simulink model "generic_20231123_1032"  (R2022b)
settings: Solver=ode45  StartTime=0.0  StopTime=50  RelTol=1e-3  EnableMultiTasking=on
model workspace (MAT data in the model file):
  A = 1
  B = 1.19071237887
  kd = -9.99955278144
  ki = 0.00519416981022
  kp = 9.99999979837
undefined symbols (not defined in the file): brake_select, curvature, DiscIntNeverNeededParam, speed
libraries: CarMaker4SL x88, simulink x1, mpcadaslib x1
(part 3 of 4)

== system generic_20231123_1032/CarMaker/IPG Vehicle/CarAndTrailer/Trailer/CreateBus Car.Hitch.FrcTrq ==
  In1 : Inport
  Bus Creator7 : BusCreator  Inputs=6
  Demux7 : Demux  Outputs=6
      settings: DisplayOption=none
  Out1 : Outport  VectorParamsAs1DForOutWhenUnconnected=off
  wires:
  In1/1 -> Demux7/1
  Bus Creator7/1 -> Out1/1
  Demux7/6 -> Bus Creator7/6  "Car Hitch Trq2Car z"
  Demux7/5 -> Bus Creator7/5  "Car Hitch Trq2Car y"
  Demux7/4 -> Bus Creator7/4  "Car Hitch Trq2Car x"
  Demux7/3 -> Bus Creator7/3  "Car Hitch Frc2Car z"
  Demux7/2 -> Bus Creator7/2  "Car Hitch Frc2Car y"
  Demux7/1 -> Bus Creator7/1  "Car Hitch Frc2Car x"

== system generic_20231123_1032/CarMaker/IPG Vehicle/CarAndTrailer/Trailer/CreateBus Vhcl.Motion ==
  In1 : Inport
  BusCreator : BusCreator  Inputs=15
  Demux : Demux  Outputs=15
      settings: DisplayOption=none
  Out1 : Outport  VectorParamsAs1DForOutWhenUnconnected=off
  wires:
  Demux/15 -> BusCreator/15  "Vhcl YawAcc"
  Demux/14 -> BusCreator/14  "Vhcl YawVel"
  Demux/13 -> BusCreator/13  "Vhcl Yaw"
  Demux/12 -> BusCreator/12  "Vhcl PitchAcc"
  Demux/11 -> BusCreator/11  "Vhcl PitchVel"
  Demux/10 -> BusCreator/10  "Vhcl Pitch"
  Demux/9 -> BusCreator/9  "Vhcl RollAcc"
  Demux/8 -> BusCreator/8  "Vhcl RollVel"
  Demux/7 -> BusCreator/7  "Vhcl Roll"
  Demux/6 -> BusCreator/6  "Vhcl Hitch_Pos z"
  Demux/5 -> BusCreator/5  "Vhcl Hitch_Pos y"
  Demux/4 -> BusCreator/4  "Vhcl Hitch_Pos x"
  Demux/3 -> BusCreator/3  "Vhcl sRoad"
  Demux/2 -> BusCreator/2  "Vhcl Distance"
  Demux/1 -> BusCreator/1  "Vhcl v"
  In1/1 -> Demux/1
  BusCreator/1 -> Out1/1

== system generic_20231123_1032/CarMaker/IPG Vehicle/CarAndTrailer/Trailer/CreateBus Vhcl.PoI ==
  In1 : Inport
  Bus Creator3 : BusCreator  Inputs=18
  Demux3 : Demux  Outputs=18
      settings: DisplayOption=none
  Out1 : Outport  VectorParamsAs1DForOutWhenUnconnected=off
  wires:
  Demux3/18 -> Bus Creator3/18  "Vhcl PoI_GCS Elev"
  Demux3/17 -> Bus Creator3/17  "Vhcl PoI_GCS Lat"
  Demux3/16 -> Bus Creator3/16  "Vhcl PoI_GCS Long"
  Demux3/15 -> Bus Creator3/15  "Vhcl PoI_Acc_1 z"
  Demux3/14 -> Bus Creator3/14  "Vhcl PoI_Acc_1 y"
  Demux3/13 -> Bus Creator3/13  "Vhcl PoI_Acc_1 x"
  Demux3/12 -> Bus Creator3/12  "Vhcl PoI_Vel_1 z"
  Demux3/11 -> Bus Creator3/11  "Vhcl PoI_Vel_1 y"
  Demux3/10 -> Bus Creator3/10  "Vhcl PoI_Vel_1 x"
  Demux3/9 -> Bus Creator3/9  "Vhcl PoI_Acc z"
  Demux3/8 -> Bus Creator3/8  "Vhcl PoI_Acc y"
  Demux3/7 -> Bus Creator3/7  "Vhcl PoI_Acc x"
  Demux3/6 -> Bus Creator3/6  "Vhcl PoI_Vel z"
  Demux3/5 -> Bus Creator3/5  "Vhcl PoI_Vel y"
  Demux3/4 -> Bus Creator3/4  "Vhcl PoI_Vel x"
  Demux3/3 -> Bus Creator3/3  "Vhcl PoI_Pos z"
  Demux3/2 -> Bus Creator3/2  "Vhcl PoI_Pos y"
  In1/1 -> Demux3/1
  Bus Creator3/1 -> Out1/1
  Demux3/1 -> Bus Creator3/1  "Vhcl PoI_Pos x"

== system generic_20231123_1032/CarMaker/IPG Vehicle/CarAndTrailer/Trailer/CreateBus Vhcl.Steering ==
  In1 : Inport
  Bus Creator3 : BusCreator  Inputs=4
  Demux : Demux
      settings: DisplayOption=none
  Out1 : Outport  VectorParamsAs1DForOutWhenUnconnected=off
  wires:
  Bus Creator3/1 -> Out1/1
  Demux/1 -> Bus Creator3/1  "Vhcl Steering Ang"
  Demux/3 -> Bus Creator3/3  "Vhcl Steering AngAcc"
  Demux/2 -> Bus Creator3/2  "Vhcl Steering AngVel"
  Demux/4 -> Bus Creator3/4  "Vhcl Steering Trq"
  In1/1 -> Demux/1

== system generic_20231123_1032/CarMaker/IPG Vehicle/CarAndTrailer/Trailer/CreateBus Vhcl.Wheel.FL ==
  In1 : Inport
  Bus Creator3 : BusCreator  Inputs=14
  Demux3 : Demux  Outputs=14
      settings: DisplayOption=none
  Out1 : Outport  VectorParamsAs1DForOutWhenUnconnected=off
  wires:
  Demux3/14 -> Bus Creator3/14  "Vhcl Wheel FL Trq_WhlBearing"
  Demux3/13 -> Bus Creator3/13  "Vhcl Wheel FL Trq_T2W"
  Demux3/12 -> Bus Creator3/12  "Vhcl Wheel FL SideSlip"
  Demux3/11 -> Bus Creator3/11  "Vhcl Wheel FL LongSlip"
  Demux3/10 -> Bus Creator3/10  "Vhcl Wheel FL vBelt"
  Demux3/9 -> Bus Creator3/9  "Vhcl Wheel FL Fz"
  Demux3/8 -> Bus Creator3/8  "Vhcl Wheel FL Fy"
  Demux3/7 -> Bus Creator3/7  "Vhcl Wheel FL Fx"
  Demux3/6 -> Bus Creator3/6  "Vhcl Wheel FL r_zxy z"
  Demux3/5 -> Bus Creator3/5  "Vhcl Wheel FL r_zxy y"
  Demux3/4 -> Bus Creator3/4  "Vhcl Wheel FL r_zxy x"
  Demux3/3 -> Bus Creator3/3  "Vhcl Wheel FL t z"
  Demux3/2 -> Bus Creator3/2  "Vhcl Wheel FL t y"
  In1/1 -> Demux3/1
  Bus Creator3/1 -> Out1/1
  Demux3/1 -> Bus Creator3/1  "Vhcl Wheel FL t x"

== system generic_20231123_1032/CarMaker/IPG Vehicle/CarAndTrailer/Trailer/CreateBus Vhcl.Wheel.FR ==
  In1 : Inport
  Bus Creator3 : BusCreator  Inputs=14
  Demux3 : Demux  Outputs=14
      settings: DisplayOption=none
  Out1 : Outport  VectorParamsAs1DForOutWhenUnconnected=off
  wires:
  Demux3/14 -> Bus Creator3/14  "Vhcl Wheel FR Trq_WhlBearing"
  Demux3/13 -> Bus Creator3/13  "Vhcl Wheel FR Trq_T2W"
  Demux3/12 -> Bus Creator3/12  "Vhcl Wheel FR SideSlip"
  Demux3/11 -> Bus Creator3/11  "Vhcl Wheel FR LongSlip"
  Demux3/10 -> Bus Creator3/10  "Vhcl Wheel FR vBelt"
  Demux3/9 -> Bus Creator3/9  "Vhcl Wheel FR Fz"
  Demux3/8 -> Bus Creator3/8  "Vhcl Wheel FR Fy"
  Demux3/7 -> Bus Creator3/7  "Vhcl Wheel FR Fx"
  Demux3/6 -> Bus Creator3/6  "Vhcl Wheel FR r_zxy z"
  Demux3/5 -> Bus Creator3/5  "Vhcl Wheel FR r_zxy y"
  Demux3/4 -> Bus Creator3/4  "Vhcl Wheel FR r_zxy x"
  Demux3/3 -> Bus Creator3/3  "Vhcl Wheel FR t z"
  Demux3/2 -> Bus Creator3/2  "Vhcl Wheel FR t y"
  In1/1 -> Demux3/1
  Bus Creator3/1 -> Out1/1
  Demux3/1 -> Bus Creator3/1  "Vhcl Wheel FR t x"

== system generic_20231123_1032/CarMaker/IPG Vehicle/CarAndTrailer/Trailer/CreateBus Vhcl.Wheel.RL ==
  In1 : Inport
  Bus Creator3 : BusCreator  Inputs=14
  Demux3 : Demux  Outputs=14
      settings: DisplayOption=none
  Out1 : Outport  VectorParamsAs1DForOutWhenUnconnected=off
  wires:
  Demux3/14 -> Bus Creator3/14  "Vhcl Wheel RL Trq_WhlBearing"
  Demux3/13 -> Bus Creator3/13  "Vhcl Wheel RL Trq_T2W"
  Demux3/12 -> Bus Creator3/12  "Vhcl Wheel RL SideSlip"
  Demux3/11 -> Bus Creator3/11  "Vhcl Wheel RL LongSlip"
  Demux3/10 -> Bus Creator3/10  "Vhcl Wheel RL vBelt"
  Demux3/9 -> Bus Creator3/9  "Vhcl Wheel RL Fz"
  Demux3/8 -> Bus Creator3/8  "Vhcl Wheel RL Fy"
  Demux3/7 -> Bus Creator3/7  "Vhcl Wheel RL Fx"
  Demux3/6 -> Bus Creator3/6  "Vhcl Wheel RL r_zxy z"
  Demux3/5 -> Bus Creator3/5  "Vhcl Wheel RL r_zxy y"
  Demux3/4 -> Bus Creator3/4  "Vhcl Wheel RL r_zxy x"
  Demux3/3 -> Bus Creator3/3  "Vhcl Wheel RL t z"
  Demux3/2 -> Bus Creator3/2  "Vhcl Wheel RL t y"
  In1/1 -> Demux3/1
  Bus Creator3/1 -> Out1/1
  Demux3/1 -> Bus Creator3/1  "Vhcl Wheel RL t x"

== system generic_20231123_1032/CarMaker/IPG Vehicle/CarAndTrailer/Trailer/CreateBus Vhcl.Wheel.RR ==
  In1 : Inport
  Bus Creator3 : BusCreator  Inputs=14
  Demux3 : Demux  Outputs=14
      settings: DisplayOption=none
  Out1 : Outport  VectorParamsAs1DForOutWhenUnconnected=off
  wires:
  Demux3/14 -> Bus Creator3/14  "Vhcl Wheel RR Trq_WhlBearing"
  Demux3/13 -> Bus Creator3/13  "Vhcl Wheel RR Trq_T2W"
  Demux3/12 -> Bus Creator3/12  "Vhcl Wheel RR SideSlip"
  Demux3/11 -> Bus Creator3/11  "Vhcl Wheel RR LongSlip"
  Demux3/10 -> Bus Creator3/10  "Vhcl Wheel RR vBelt"
  Demux3/9 -> Bus Creator3/9  "Vhcl Wheel RR Fz"
  Demux3/8 -> Bus Creator3/8  "Vhcl Wheel RR Fy"
  Demux3/7 -> Bus Creator3/7  "Vhcl Wheel RR Fx"
  Demux3/6 -> Bus Creator3/6  "Vhcl Wheel RR r_zxy z"
  Demux3/5 -> Bus Creator3/5  "Vhcl Wheel RR r_zxy y"
  Demux3/4 -> Bus Creator3/4  "Vhcl Wheel RR r_zxy x"
  Demux3/3 -> Bus Creator3/3  "Vhcl Wheel RR t z"
  Demux3/2 -> Bus Creator3/2  "Vhcl Wheel RR t y"
  In1/1 -> Demux3/1
  Bus Creator3/1 -> Out1/1
  Demux3/1 -> Bus Creator3/1  "Vhcl Wheel RR t x"

== system generic_20231123_1032/CarMaker/VehicleControl/CreateBus VhclCtrl/Stanley_controller/Stanley ==
  Path_out : Inport
  <Vx_Global_m_s> : Inport  Port=2
  <Vy_Global_m_s> : Inport  Port=3
  <Yaw_angle_rad> : Inport  Port=4
  <Actual_Velocity_Car_m_s> : Inport  Port=5
  Desired_speed : Inport  Port=6
  Actual velocity [km/h] : Display
  Bus Selector : BusSelector  OutputSignals=Path.tx,Path.ty
  Constant1 : Constant  Value=0
  Delay : Delay  DelayLength=1
  Delay1 : Delay  DelayLength=1
  Gain : Gain  Gain=3.6
  Read CM Dict : CarMaker4SL/Read CM Dict  xname=Car.Road.Path.DevDist  xsync=off  xstime=Continuous
  Read CM Dict1 : CarMaker4SL/Read CM Dict  xname=Car.Con.tx  xsync=off  xstime=Continuous
  Read CM Dict2 : CarMaker4SL/Read CM Dict  xname=Car.Con.ty  xsync=off  xstime=Continuous
  Road Sensor : CarMaker4SL/Sensors/Road Sensor  xname=0  xstime=Continuous
      settings: SourceProductName=CarMaker4SL
  Saturation : Saturate  UpperLimit=pi()/6  LowerLimit=-pi/6
  Scope : Scope  NumInputPorts=3
  Smoothing : Subsystem
  Stanely_controller : MATLAB Function  TreatAsAtomicUnit=on
  Subsystem : Subsystem
  Subsystem1 : Subsystem
  Target_Steering_angle_rad : Outport  VectorParamsAs1DForOutWhenUnconnected=off
  Throttle : Outport  Port=2
  Brake_command : Outport  Port=3
  wires:
  Smoothing/1(Signal_Out) -> Target_Steering_angle_rad/1, Scope/3
  Saturation/1 -> Smoothing/1(Signal_In)  "Control signal"
  Subsystem/4(min_safe_speed) -> Subsystem1/3(min_safe_speed)
  Subsystem/2(Brake_command) -> Brake_command/1
  Subsystem/3(path_curvature) -> Subsystem1/2(curvature)
  Gain/1 -> Actual velocity [km/h]/1  "Actual velocity [km/h]"
  Stanely_controller/1(e) -> Scope/1  "Control cross track error [m]"
  <Actual_Velocity_Car_m_s>/1 -> Gain/1, Subsystem/2(speed_act), Stanely_controller/8(speed_act)
  Subsystem1/1(Target_speed) -> Subsystem/5(desired_speed)
  <Vx_Global_m_s>/1 -> Subsystem/3(velocity_x)
  <Vy_Global_m_s>/1 -> Subsystem/4(velocity_y)
  Path_out/1 -> Subsystem/1(path)
  Desired_speed/1 -> Subsystem1/1(desired_speed)
  Stanely_controller/7(steering) -> Subsystem/6(steering), Saturation/1  "steering"
  Subsystem/1(Throttle) -> Throttle/1
  Stanely_controller/6(heading_err) -> ?  "heading_error"
  Stanely_controller/2(a) -> ?  "Error [m]"
  Stanely_controller/3(b) -> ?
  Bus Selector/1 -> Stanely_controller/4(x2), Delay/1  "<tx>"
  Constant1/1 -> Road Sensor/1
  Road Sensor/2 -> Bus Selector/1
  Bus Selector/2 -> Stanely_controller/6(y2), Delay1/1  "<ty>"
  Delay1/1 -> Stanely_controller/5(y1)
  <Yaw_angle_rad>/1 -> Stanely_controller/7(yaw)  "Yaw [rad]"
  Delay/1 -> Stanely_controller/3(x1)
  Read CM Dict1/1 -> Stanely_controller/1(x_car)
  Read CM Dict/1 -> Stanely_controller/2(dev), Scope/2  "Dev_dis"

== system generic_20231123_1032/CarMaker/VehicleControl/CreateBus VhclCtrl/Subsystem1/Smoothing ==
  Signal_In : Inport
  Add : Sum  Inputs=++++
  Delay : Delay  InitialCondition=0.1
  Delay1 : Delay  DelayLength=4  InitialCondition=0.1
  Delay2 : Delay  DelayLength=5  InitialCondition=0.1
  Gain : Gain  Gain=0.35
  Gain1 : Gain  Gain=0.25
  Gain2 : Gain  Gain=0.25
  Gain3 : Gain  Gain=0.15
  Signal_Out : Outport  VectorParamsAs1DForOutWhenUnconnected=off
  wires:
  Gain1/1 -> Add/2
  Signal_In/1 -> Gain/1
  Delay/1 -> Gain1/1
  Gain/1 -> Add/1
  Delay1/1 -> Gain2/1
  Add/1 -> Delay2/1, Delay1/1, Delay/1, Signal_Out/1
  Gain2/1 -> Add/3
  Delay2/1 -> Gain3/1
  Gain3/1 -> Add/4

== system generic_20231123_1032/CarMaker/VehicleControl/CreateBus VhclCtrl/Subsystem4/Subsystem ==
  In1 : Inport
  Add : Sum  Inputs=+++
  Derivative : Derivative
  Discrete-Time Integrator : DiscreteIntegrator  SampleTime=-1  ICPrevOutput=DiscIntNeverNeededParam  ICPrevScaledInput=DiscIntNeverNeededParam
  Gain : Gain  Gain=0.6
  Gain1 : Gain  Gain=1.2
  Gain2 : Gain  Gain=0.4
  Signal_In : Outport
  wires:
  Gain1/1 -> Discrete-Time Integrator/1
  Gain2/1 -> Derivative/1
  Discrete-Time Integrator/1 -> Add/1
  Derivative/1 -> Add/3
  Gain/1 -> Add/2
  In1/1 -> Gain/1, Gain2/1, Gain1/1
  Add/1 -> Signal_In/1

== system generic_20231123_1032/CarMaker/VehicleControl/CreateBus VhclCtrl/path_planner_MATLAB/X_Global_Pos_m ==
  In1 : Inport
  Pos_X : Outport  VectorParamsAs1DForOutWhenUnconnected=off
  wires:
  In1/1 -> Pos_X/1

== system generic_20231123_1032/CarMaker/VehicleControl/CreateBus VhclCtrl/path_planner_MATLAB/Y_Global_Pos_m ==
  In1 : Inport
  Pos_Y : Outport  VectorParamsAs1DForOutWhenUnconnected=off
  wires:
  In1/1 -> Pos_Y/1

== system generic_20231123_1032/CarMaker/VehicleControl/CreateBus VhclCtrl/path_planner_MATLAB/Yaw_angle_rad ==
  In1 : Inport
  Yaw_Angle : Outport  VectorParamsAs1DForOutWhenUnconnected=off
  wires:
  In1/1 -> Yaw_Angle/1

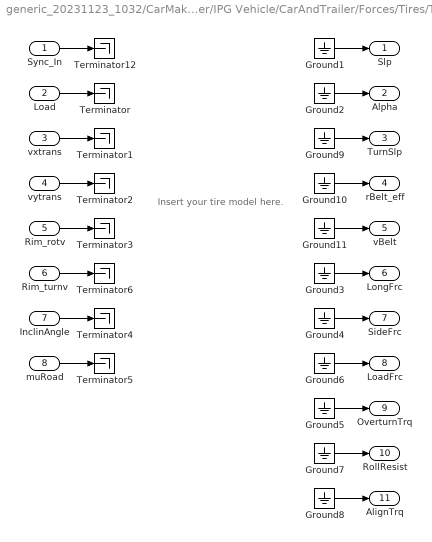
== system generic_20231123_1032/CarMaker/IPG Vehicle/CarAndTrailer/Forces/Tires/TireFL ==
  note: Insert your tire model here.
  Sync_In : Inport
  Load : Inport  Port=2
  vxtrans : Inport  Port=3
  vytrans : Inport  Port=4
  Rim_rotv : Inport  Port=5
  Rim_turnv : Inport  Port=6
  InclinAngle : Inport  Port=7
  muRoad : Inport  Port=8
  Ground{1..11} (11 alike) : Ground
  Terminator{,1..6,12} (8 alike) : Terminator
  Slp : Outport  VectorParamsAs1DForOutWhenUnconnected=off
  Alpha : Outport  Port=2  VectorParamsAs1DForOutWhenUnconnected=off
  TurnSlp : Outport  Port=3  VectorParamsAs1DForOutWhenUnconnected=off
  rBelt_eff : Outport  Port=4  VectorParamsAs1DForOutWhenUnconnected=off
  vBelt : Outport  Port=5  VectorParamsAs1DForOutWhenUnconnected=off
  LongFrc : Outport  Port=6  VectorParamsAs1DForOutWhenUnconnected=off
  SideFrc : Outport  Port=7  VectorParamsAs1DForOutWhenUnconnected=off
  LoadFrc : Outport  Port=8  VectorParamsAs1DForOutWhenUnconnected=off
  OverturnTrq : Outport  Port=9  VectorParamsAs1DForOutWhenUnconnected=off
  RollResist : Outport  Port=10  VectorParamsAs1DForOutWhenUnconnected=off
  AlignTrq : Outport  Port=11  VectorParamsAs1DForOutWhenUnconnected=off
  wires:
  Ground11/1 -> vBelt/1
  Ground10/1 -> rBelt_eff/1
  Ground9/1 -> TurnSlp/1
  Rim_turnv/1 -> Terminator6/1
  Sync_In/1 -> Terminator12/1
  Ground2/1 -> Alpha/1
  Ground3/1 -> LongFrc/1
  Ground4/1 -> SideFrc/1
  Ground5/1 -> OverturnTrq/1
  vxtrans/1 -> Terminator1/1
  vytrans/1 -> Terminator2/1
  Rim_rotv/1 -> Terminator3/1
  InclinAngle/1 -> Terminator4/1
  muRoad/1 -> Terminator5/1
  Load/1 -> Terminator/1
  Ground1/1 -> Slp/1
  Ground6/1 -> LoadFrc/1
  Ground7/1 -> RollResist/1
  Ground8/1 -> AlignTrq/1

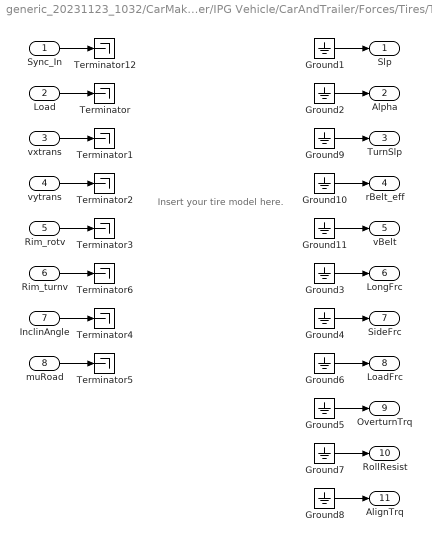
== system generic_20231123_1032/CarMaker/IPG Vehicle/CarAndTrailer/Forces/Tires/TireFR ==
  note: Insert your tire model here.
  Sync_In : Inport
  Load : Inport  Port=2
  vxtrans : Inport  Port=3
  vytrans : Inport  Port=4
  Rim_rotv : Inport  Port=5
  Rim_turnv : Inport  Port=6
  InclinAngle : Inport  Port=7
  muRoad : Inport  Port=8
  Ground{1..11} (11 alike) : Ground
  Terminator{,1..6,12} (8 alike) : Terminator
  Slp : Outport  VectorParamsAs1DForOutWhenUnconnected=off
  Alpha : Outport  Port=2  VectorParamsAs1DForOutWhenUnconnected=off
  TurnSlp : Outport  Port=3  VectorParamsAs1DForOutWhenUnconnected=off
  rBelt_eff : Outport  Port=4  VectorParamsAs1DForOutWhenUnconnected=off
  vBelt : Outport  Port=5  VectorParamsAs1DForOutWhenUnconnected=off
  LongFrc : Outport  Port=6  VectorParamsAs1DForOutWhenUnconnected=off
  SideFrc : Outport  Port=7  VectorParamsAs1DForOutWhenUnconnected=off
  LoadFrc : Outport  Port=8  VectorParamsAs1DForOutWhenUnconnected=off
  OverturnTrq : Outport  Port=9  VectorParamsAs1DForOutWhenUnconnected=off
  RollResist : Outport  Port=10  VectorParamsAs1DForOutWhenUnconnected=off
  AlignTrq : Outport  Port=11  VectorParamsAs1DForOutWhenUnconnected=off
  wires:
  Ground11/1 -> vBelt/1
  Ground10/1 -> rBelt_eff/1
  Ground9/1 -> TurnSlp/1
  Rim_turnv/1 -> Terminator6/1
  Sync_In/1 -> Terminator12/1
  Ground2/1 -> Alpha/1
  Ground3/1 -> LongFrc/1
  Ground4/1 -> SideFrc/1
  Ground5/1 -> OverturnTrq/1
  vxtrans/1 -> Terminator1/1
  vytrans/1 -> Terminator2/1
  Rim_rotv/1 -> Terminator3/1
  InclinAngle/1 -> Terminator4/1
  muRoad/1 -> Terminator5/1
  Load/1 -> Terminator/1
  Ground1/1 -> Slp/1
  Ground6/1 -> LoadFrc/1
  Ground7/1 -> RollResist/1
  Ground8/1 -> AlignTrq/1

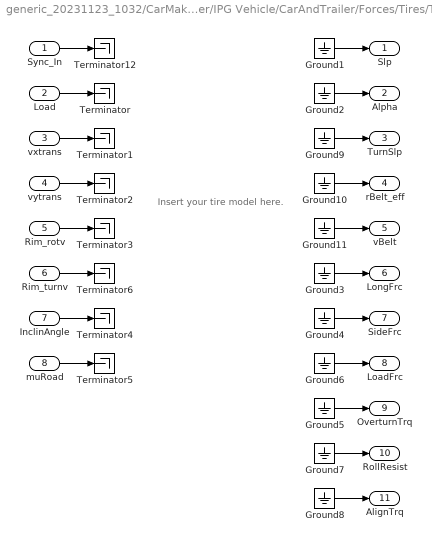
== system generic_20231123_1032/CarMaker/IPG Vehicle/CarAndTrailer/Forces/Tires/TireRL ==
  note: Insert your tire model here.
  Sync_In : Inport
  Load : Inport  Port=2
  vxtrans : Inport  Port=3
  vytrans : Inport  Port=4
  Rim_rotv : Inport  Port=5
  Rim_turnv : Inport  Port=6
  InclinAngle : Inport  Port=7
  muRoad : Inport  Port=8
  Ground{1..11} (11 alike) : Ground
  Terminator{,1..6,12} (8 alike) : Terminator
  Slp : Outport  VectorParamsAs1DForOutWhenUnconnected=off
  Alpha : Outport  Port=2  VectorParamsAs1DForOutWhenUnconnected=off
  TurnSlp : Outport  Port=3  VectorParamsAs1DForOutWhenUnconnected=off
  rBelt_eff : Outport  Port=4  VectorParamsAs1DForOutWhenUnconnected=off
  vBelt : Outport  Port=5  VectorParamsAs1DForOutWhenUnconnected=off
  LongFrc : Outport  Port=6  VectorParamsAs1DForOutWhenUnconnected=off
  SideFrc : Outport  Port=7  VectorParamsAs1DForOutWhenUnconnected=off
  LoadFrc : Outport  Port=8  VectorParamsAs1DForOutWhenUnconnected=off
  OverturnTrq : Outport  Port=9  VectorParamsAs1DForOutWhenUnconnected=off
  RollResist : Outport  Port=10  VectorParamsAs1DForOutWhenUnconnected=off
  AlignTrq : Outport  Port=11  VectorParamsAs1DForOutWhenUnconnected=off
  wires:
  Ground11/1 -> vBelt/1
  Ground10/1 -> rBelt_eff/1
  Ground9/1 -> TurnSlp/1
  Rim_turnv/1 -> Terminator6/1
  Sync_In/1 -> Terminator12/1
  Ground2/1 -> Alpha/1
  Ground3/1 -> LongFrc/1
  Ground4/1 -> SideFrc/1
  Ground5/1 -> OverturnTrq/1
  vxtrans/1 -> Terminator1/1
  vytrans/1 -> Terminator2/1
  Rim_rotv/1 -> Terminator3/1
  InclinAngle/1 -> Terminator4/1
  muRoad/1 -> Terminator5/1
  Load/1 -> Terminator/1
  Ground1/1 -> Slp/1
  Ground6/1 -> LoadFrc/1
  Ground7/1 -> RollResist/1
  Ground8/1 -> AlignTrq/1

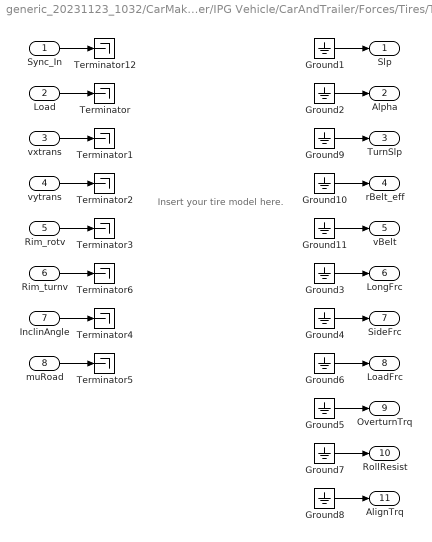
== system generic_20231123_1032/CarMaker/IPG Vehicle/CarAndTrailer/Forces/Tires/TireRR ==
  note: Insert your tire model here.
  Sync_In : Inport
  Load : Inport  Port=2
  vxtrans : Inport  Port=3
  vytrans : Inport  Port=4
  Rim_rotv : Inport  Port=5
  Rim_turnv : Inport  Port=6
  InclinAngle : Inport  Port=7
  muRoad : Inport  Port=8
  Ground{1..11} (11 alike) : Ground
  Terminator{,1..6,12} (8 alike) : Terminator
  Slp : Outport  VectorParamsAs1DForOutWhenUnconnected=off
  Alpha : Outport  Port=2  VectorParamsAs1DForOutWhenUnconnected=off
  TurnSlp : Outport  Port=3  VectorParamsAs1DForOutWhenUnconnected=off
  rBelt_eff : Outport  Port=4  VectorParamsAs1DForOutWhenUnconnected=off
  vBelt : Outport  Port=5  VectorParamsAs1DForOutWhenUnconnected=off
  LongFrc : Outport  Port=6  VectorParamsAs1DForOutWhenUnconnected=off
  SideFrc : Outport  Port=7  VectorParamsAs1DForOutWhenUnconnected=off
  LoadFrc : Outport  Port=8  VectorParamsAs1DForOutWhenUnconnected=off
  OverturnTrq : Outport  Port=9  VectorParamsAs1DForOutWhenUnconnected=off
  RollResist : Outport  Port=10  VectorParamsAs1DForOutWhenUnconnected=off
  AlignTrq : Outport  Port=11  VectorParamsAs1DForOutWhenUnconnected=off
  wires:
  Ground11/1 -> vBelt/1
  Ground10/1 -> rBelt_eff/1
  Ground9/1 -> TurnSlp/1
  Rim_turnv/1 -> Terminator6/1
  Sync_In/1 -> Terminator12/1
  Ground2/1 -> Alpha/1
  Ground3/1 -> LongFrc/1
  Ground4/1 -> SideFrc/1
  Ground5/1 -> OverturnTrq/1
  vxtrans/1 -> Terminator1/1
  vytrans/1 -> Terminator2/1
  Rim_rotv/1 -> Terminator3/1
  InclinAngle/1 -> Terminator4/1
  muRoad/1 -> Terminator5/1
  Load/1 -> Terminator/1
  Ground1/1 -> Slp/1
  Ground6/1 -> LoadFrc/1
  Ground7/1 -> RollResist/1
  Ground8/1 -> AlignTrq/1

== system generic_20231123_1032/CarMaker/VehicleControl/CreateBus VhclCtrl/Stanley_controller/Stanley/Smoothing ==
  Signal_In : Inport
  Add : Sum  Inputs=++++
  Delay : Delay  InitialCondition=0.1
  Delay1 : Delay  DelayLength=4  InitialCondition=0.1
  Delay2 : Delay  DelayLength=5  InitialCondition=0.1
  Gain : Gain  Gain=0.35
  Gain1 : Gain  Gain=0.25
  Gain2 : Gain  Gain=0.25
  Gain3 : Gain  Gain=0.15
  Signal_Out : Outport  VectorParamsAs1DForOutWhenUnconnected=off
  wires:
  Gain1/1 -> Add/2
  Signal_In/1 -> Gain/1
  Delay/1 -> Gain1/1
  Gain/1 -> Add/1
  Delay1/1 -> Gain2/1
  Add/1 -> Delay2/1, Delay1/1, Delay/1, Signal_Out/1
  Gain2/1 -> Add/3
  Delay2/1 -> Gain3/1
  Gain3/1 -> Add/4

== system generic_20231123_1032/CarMaker/VehicleControl/CreateBus VhclCtrl/Stanley_controller/Stanley/Subsystem ==
  path : Inport
  speed_act : Inport  Port=2
  velocity_x : Inport  Port=3
  velocity_y : Inport  Port=4
  desired_speed : Inport  Port=5
  steering : Inport  Port=6
  Constant : Constant  Value=0
  Constant1 : Constant  Value=kd
  Constant2 : Constant  Value=ki
  Constant3 : Constant  Value=kp
  Gain : Gain  Gain=1/1000
  Gain1 : Gain  Gain=1/1000
  Saturation : Saturate  UpperLimit=1  LowerLimit=-1
  Saturation1 : Saturate  UpperLimit=1  LowerLimit=0
  Scope : Scope  NumInputPorts=2
  advanced_speed_and_brake_control : MATLAB Function  TreatAsAtomicUnit=on
  calculate_path_curvature : MATLAB Function  TreatAsAtomicUnit=on
  Throttle : Outport
  Brake_command : Outport  Port=2
  path_curvature : Outport  Port=3
  min_safe_speed : Outport  Port=4
  wires:
  Saturation/1 -> Scope/2, Throttle/1
  Saturation1/1 -> Brake_command/1  "Brake_command"
  advanced_speed_and_brake_control/2(brake_cmd) -> Gain1/1  "Brake cmd"
  advanced_speed_and_brake_control/1(throttle) -> Gain/1  "throttle"
  desired_speed/1 -> advanced_speed_and_brake_control/4(desired_speed)
  speed_act/1 -> advanced_speed_and_brake_control/3(speed_act)
  Constant/1 -> advanced_speed_and_brake_control/1(path_curv)
  calculate_path_curvature/2(min_safe_speed) -> min_safe_speed/1, advanced_speed_and_brake_control/2(min_s_speed)
  steering/1 -> calculate_path_curvature/4(steering_angel)
  calculate_path_curvature/1(path_curvature) -> path_curvature/1
  velocity_x/1 -> calculate_path_curvature/3(velocity_x)
  velocity_y/1 -> calculate_path_curvature/2(velocity_y)
  path/1 -> calculate_path_curvature/1(path)
  Gain/1 -> Scope/1, Saturation/1
  Gain1/1 -> Saturation1/1
  Constant1/1 -> advanced_speed_and_brake_control/5(Kd_speed)
  Constant2/1 -> advanced_speed_and_brake_control/6(Ki_speed)
  Constant3/1 -> advanced_speed_and_brake_control/7(Kp_speed)

== system generic_20231123_1032/CarMaker/VehicleControl/CreateBus VhclCtrl/Stanley_controller/Stanley/Subsystem1 ==
  desired_speed : Inport
  curvature : Inport  Port=2
  min_safe_speed : Inport  Port=3
  2-D Lookup Table : Lookup_n-D  BreakpointsForDimension1=speed  BreakpointsForDimension2=curvature  Table=brake_select  InternalRulePriority=Speed  RndMeth=Simplest
      settings: InputPortMap=u0,u1
  Divide : Product  Inputs=*/
  MATLAB Function : MATLAB Function  Commented=on  TreatAsAtomicUnit=on
  Read CM Dict : CarMaker4SL/Read CM Dict  xname=Sensor.Road.VehSensor_0.Path.CurveXY  xsync=off  xstime=Continuous
  Scope2 : Scope
  Target_speed : Outport
  curv : Outport  Port=2
  speed : Outport  Port=3
  wires:
  Divide/1 -> speed/1, Target_speed/1, Scope2/1
  2-D Lookup Table/1 -> Divide/2
  desired_speed/1 -> 2-D Lookup Table/1, Divide/1
  min_safe_speed/1 -> MATLAB Function/2(min_safe_speed)
  curvature/1 -> MATLAB Function/1(u)
  Read CM Dict/1 -> curv/1, 2-D Lookup Table/2

== matlab function generic_20231123_1032/CarMaker/VehicleControl/Stanley controller/calculate_path_curvature ==
  data: path_x input; path_curvature output; path_y input
function path_curvature = calculate_path_curvature(path_x,path_y)
    x = path_x;
    y = path_y;
    % First and second derivatives
    dx = gradient(x);
    dy = gradient(y);
    
    ddx = gradient(dx);
    ddy = gradient(dy);
    
    % Path curvature
    path_curvature = mean((dx .* ddy - dy .* ddx) ./ (dx.^2 + dy.^2).^(3/2));
    %R = sqrt(1.61^2 +(1.61+1.28)^2*cot(steering_angel)^2)/12;
    
end

== matlab function generic_20231123_1032/CarMaker/VehicleControl/Stanley controller/MATLAB Function ==
  data: path input; dev input; e output; yaw input; speed_act input; err_fr_axle output; cross_track_steering output; heading_err output; steering output
function [e, err_fr_axle, cross_track_steering, heading_err, steering]  = conversion(path,dev,yaw,speed_act)
%path = [path_x;path_y];
function distance = calc_distance(pt,v1,v2)
    vect = v1 - v2;
    p_to_vect = pt - v2;
    crossVP = cross(vect,p_to_vect);
    distance = norm(crossVP) / norm(vect) * crossVP(3)/abs(crossVP(3));
end

e = zeros(1);
cross_track_steering = zeros(1);
heading_err = zeros(1);
steering=zeros(1);
err_fr_axle = zeros(1);

k_exp = 1.3059;
k = 15.028 + speed_act^k_exp;
k_ref = 2.62;

% path_index = fix(k_path * speed_act);
% if path_index > 13
%     path_index = 13;
% end
% 
% P_prev = path(:,6 + path_index);
% P_next = path(:,7 + path_index);

fr_axle = [-1.488 0 0];
distances = sqrt((path(1,:) - 1.488).^2 + (path(2,:) - 0).^2);
% Find the index of the closest point on the path
[~,err_fr_axle_ind] = min(distances);
if err_fr_axle_ind == 1
    err_fr_axle_ind = 2;
end
err_fr_axle = calc_distance(fr_axle,[path(1,err_fr_axle_ind - 1) path(2,err_fr_axle_ind - 1) 0],[path(1,err_fr_axle_ind) path(2,err_fr_axle_ind) 0]);

B = [-1.488 + k_ref * (speed_act / 27) 0 0];
distances_err = sqrt((path(1,:) - B(1)).^2 + (path(2,:) - 0).^2);
[~,err_ind] = min(distances_err);
if err_ind < 2
    err_ind = 2;
end
error = calc_distance(B,[path(1,err_ind - 1) path(2,err_ind - 1) 0],[path(1,err_ind) path(2,err_ind) 0]);


P_prev = path(:, err_ind-1);
P_next = path(:, err_ind);

x1 = P_prev(1,1);
y1 = P_prev(2,1);
x2 = P_next(1,1);
y2 = P_next(2,1);

a = (y2 - y1)/-(x2 + x1);
b = 1;
%c = -x1 * (y2 - y1) + y1 * (x2 - x1);


if speed_act ~= 0
    %e = c+b*y1/sqrt((a^2)+(b^2));
    e = error;
    
    cross_track_steering = atan(k * e / speed_act);
    heading_err = atan(-a / b) - yaw;
    %heading_err = 1/(tan(-a/b))-yaw;
    steering = heading_err + cross_track_steering;
end
end

== matlab function generic_20231123_1032/CarMaker/VehicleControl/CreateBus VhclCtrl/Subsystem1/MATLAB Function1 ==
  data: dev input; steering output; B input
function steering = advanced_speed_control_mpc(dev,B)
    % Model Predictive Controller (MPC) for speed contol
    % Define MPC parameters
    Ts = 0.1;  % Sampling time
    N = 10;    % Prediction horizon
    Q = 1;     % State weight
    R = 1;     % Input weight
    S = 0.1;   % Terminal state weight (integral term)
    
    % State-space model (simplified for illustration)
    %A = 0.8;
    %B = Ts;
    
    % Define cost and constraints for fmincon
    costFunction = @(u) (dev + B * u)' * Q * (dev + B * u) + u' * R * u + S * sum(u);
    Aeq = [];
    Beq = [];
    Aineq = [];
    Bineq = [];
    lb = -3.14; % Lower bound on throttle
    ub = 3.14;  % Upper bound on throttle
    
    % Steady-state error constraint
    Aineq = [Aineq; B];
    Bineq = [Bineq; -dev];
    
    % Initial guess
    u0 = 0;
    
    % Solve optimization problem
    options = optimoptions('fmincon', 'Display', 'off', 'Algorithm', 'sqp');
    u_opt = fmincon(costFunction, u0, Aineq, Bineq, Aeq, Beq, lb, ub, [], options);
    
    % Extract control input (throttle) from the optimization result
    steering = u_opt;
end

== matlab function generic_20231123_1032/CarMaker/VehicleControl/CreateBus VhclCtrl/Stanley_controller/Stanley/Subsystem/calculate_path_curvature ==
  data: path input; path_curvature output size=[1 20]; min_safe_speed output size=[1 20]; velocity_y input; velocity_x input; steering_angel input
function [path_curvature, min_safe_speed] = calculate_path_curvature(path,velocity_y,velocity_x,steering_angel)
    v_x = velocity_x* ones(1,20);
    v_y = velocity_y*ones(1,20);
    x = path(1,:)+v_x;
    y = path(2,:)+v_y;
    % First and second derivatives
    dx = gradient(x);
    dy = gradient(y);
    
    ddx = gradient(dx);
    ddy = gradient(dy);
    
    % Path curvature
    path_curvature = (dx .* ddy - dy .* ddx) ./ (dx.^2 + dy.^2).^(3/2);
    R = sqrt(1.61^2 +(1.61+1.28)^2*cot(steering_angel)^2)/12;
    % Minimum safe speed
    g = 9.81; % gravitational acceleration
    if max(path_curvature)>0.001 || max(path_curvature)<-0.001

        min_safe_speed = sqrt(g ./ abs(path_curvature));
    else
        min_safe_speed = sqrt(g .* abs(path_curvature));
end

== matlab function generic_20231123_1032/CarMaker/VehicleControl/CreateBus VhclCtrl/Stanley_controller/Stanley/Stanely_controller ==
  data: x_car input; dev input; x1 input; x2 input; y1 input; y2 input; yaw input; speed_act input; e output; a output; b output; c output; cross_track_steering output; heading_err output; steering output; distances output
function [e, a,b,c, cross_track_steering, heading_err, steering,distances]  = conversion(x_car,dev, x1,x2,y1,y2,yaw,speed_act)


e = zeros(1);
cross_track_steering = zeros(1);
heading_err = zeros(1);
steering=zeros(1);
err_fr_axle = zeros(1);
distances = [0 0 0 0 0 0 0 0 0 0 0 0 0 0 0 0 0 0 0 0];

k_exp = 1.36;
k_def = 6;
k = k_def + abs(speed_act)^k_exp;
k_ref = 3.1;



% Perform linear regression to find a, b, and c
% X = [path(1, :); path(2, :); ones(1, 20)]';  % Create a matrix for linear regression
% coefficients = X \ -1 * ones(20, 1);
% 
% % Extract the coefficients a, b, and c
% a = coefficients(1);
% b = coefficients(2);
% c = coefficients(3);



%Trajectory line ax+by+c = 0
% OR y= slope *x +y_intercept
% slope = path(2,)% [2-20]
if (x2 ==0 && x1 ==0)|| x2==x1
a = 0;
b = 1;
c = y2+a*x2;
else
a = -(y2 - y1)/(x2-x1);
b = 1;
c = y2+a*x2;
end

if speed_act ~=0
    %e =abs(a*x_car+b*y_car+c)\sqrt(a^2+b^2); %abs(Dev_dis);
    e =abs(dev);
    cross_track_steering = atan(e*k / speed_act);

    heading_err = atan(-a/b)-yaw;
    steering = heading_err + cross_track_steering;

else
    steering = 0;
end
end

== matlab function generic_20231123_1032/CarMaker/VehicleControl/CreateBus VhclCtrl/Subsystem1/MATLAB Function2 ==
  data: x_car input; target_heading output; y_car input; x_path input; y_path input; yaw_angle input; current_heading output
function [target_heading, current_heading] = calculate_headings(x_car, y_car, x_path, y_path, yaw_angle)
    % Calculate headings based on car and path positions and yaw angle
    function angle = normalize_angle(angle)
    % Normalize an angle to be in the range [-pi, pi]
    while angle > pi
        angle = angle - 2*pi;
    end

    while angle < -pi
        angle = angle + 2*pi;
    end
end
    % Calculate angle from car to path (target_heading)
    target_heading = atan2(y_path - y_car, x_path - x_car);
    
    % Adjust yaw angle to be in the range [-pi, pi]
    yaw_angle = normalize_angle(yaw_angle);
    
    % Current heading is the yaw angle of the vehicle
    current_heading = yaw_angle;
end

== matlab function generic_20231123_1032/CarMaker/VehicleControl/CreateBus VhclCtrl/Stanley_controller/Stanley/Subsystem1/MATLAB Function ==
  data: u input; curv output; min_safe_speed input; speed output
function [curv, speed] = fcn(u, min_safe_speed)

curv = abs(max(u));
speed = max(min_safe_speed);

== matlab function generic_20231123_1032/CarMaker/VehicleControl/CreateBus VhclCtrl/Subsystem1/MATLAB Function3 ==
  data: target_heading input; delta output; current_heading input; dt input; vx input; vy input
function delta = adaptive_steering_mpc(target_heading, current_heading, dt,vx,vy)
    % Adaptive Model Predictive Controller (Adaptive MPC) for steering control
    function dx = calculate_dynamics(u, m, l, Iz, dt, vx, vy)
    % Calculate the dynamics of the system (Bicycle Model)

    % Unpack state variables
    vy1 = vy - l * u;  % Correct lateral velocity for the tire slip angle

    % Bicycle model equations
    a = (2 * (u - vy1)) / (m * vx);
    b = (2 * l * (u - vy1)) / Iz;

    % State dynamics
    dx1 = a * dt;
    dx2 = b * dt;

    % Update state variables
    dx = [dx1; dx2];
end
    % Define Q and R matrices
    Q = eye(2);  % Weighting matrix for state
    R = eye(1);  % Weighting matrix for control input

    % Define system parameters (replace these with your actual vehicle parameters)
    m = 1600;           % Vehicle mass [kg]
    l = 2.975;          % Wheelbase [m]
    Iz = 2986.624;      % Vehicle inertia [kg*m^2]
    
    % Adaptive parameters
    alpha = 0.1;  % Adaptation rate
    theta = [0.1; 0.1];  % Initial guess of parameters
    
    % State vector (simplified, assuming current_heading is the heading error)
    x = [current_heading; 0];
    
    % Define cost and constraints for fmincon
    costFunction = @(u) (x + calculate_dynamics(u, m, l, Iz, dt,vx,vy))' * Q * (x + calculate_dynamics(u, m, l, Iz, dt,vx,vy)) + u' * R * u;
    Aeq = [];
    Beq = [];
    Aineq = [];
    Bineq = [];
    lb = -1.6;  % Lower bound on steering input
    ub = 1.6;   % Upper bound on steering input
    
    % Initial guess
    u0 = 0.1;
    
    % Solve optimization problem to get optimal steering input
    options = optimoptions('fmincon', 'Display', 'off', 'Algorithm', 'sqp');
    u_opt = fmincon(costFunction, u0, Aineq, Bineq, Aeq, Beq, lb, ub, [], options);
    
    % Update adaptive parameters online (using a simple gradient descent)
    x_next = x + calculate_dynamics(u_opt, m, l, Iz, dt,vx,vy);
    theta = theta - alpha * (x_next - (x + calculate_dynamics(u_opt, m, l, Iz, dt,vx,vy))) * x';
    
    % Extract control input (steering angle) from the optimization result
    delta = u_opt;
end

== matlab function generic_20231123_1032/CarMaker/VehicleControl/CreateBus VhclCtrl/Subsystem1/MATLAB Function4 ==
  data: target_heading input; delta output; current_heading input; dt input
function delta = mpc_steering_control(target_heading, current_heading, dt)
    % Model Predictive Controller (MPC) for steering control
    
    % Parameters
    Ts = 0.1;  % Sampling time
    N = 10;    % Prediction horizon
    
    % System dynamics (simplified for illustration)
    A = eye(2);  % State matrix (identity matrix for simplicity)
    B = [0; 1];  % Input matrix (represents steering input)
    
    % State vector (simplified, assuming current_heading is the heading error)
    x = [current_heading; 0];
    
    % Define cost and constraints for fmincon
    costFunction = @(u) (x + A * x + B * u)' * (x + A * x + B * u);
    Aeq = [];
    Beq = [];
    Aineq = [];
    Bineq = [];
    lb = -1.5;  % Lower bound on steering input
    ub = 1.5;   % Upper bound on steering input
    
    % Initial guess
    u0 = 0;
    
    % Solve optimization problem to get optimal steering input
    options = optimoptions('fmincon', 'Display', 'off', 'Algorithm', 'sqp');
    u_opt = fmincon(costFunction, u0, Aineq, Bineq, Aeq, Beq, lb, ub, [], options);
    
    % Extract control input (steering angle) from the optimization result
    delta = u_opt;
end

== matlab function generic_20231123_1032/CarMaker/VehicleControl/Stanley controller/Path_Calculation_V02 ==
  data: x_car input; closest_point output; y_car input; path_x input; instantaneous_path output; y_path input
function [closest_point, instantaneous_path] = calculate_path(x_car, y_car, path_x, y_path)
% x_car: x position of the car
% y_car: y position of the car
% path: [2x400] matrix representing the path
path = [path_x;y_path];
%Smoothing the Path
x = path(1,:);
y = path(2,:);
% Define the number of points you want to add for interpolation
num_extra_points = 10000; % Adjust this value as per your requirements
% Compute the total number of points after interpolation
total_points = numel(x) + num_extra_points;
existing_indices = 1:numel(x);
% Create an array of indices for the interpolated points
interpolated_indices = linspace(1, numel(x), total_points);
% Perform spline interpolation on both x and y coordinates
x_interpolated = spline(existing_indices, x, interpolated_indices);
y_interpolated = spline(existing_indices, y, interpolated_indices);

smoothed_path =vertcat(x_interpolated, y_interpolated);
% smoothed_path = smoothed_path_t';


% Calculate the distance between the car and each point on the path
distances = sqrt((smoothed_path(1,:) - x_car).^2 + (smoothed_path(2,:) - y_car).^2);

% Find the index of the closest point on the path
[~, closest_index] = min(distances);

% Get the closest point on the path
closest_point = smoothed_path(:, closest_index);

% Calculate the distance from the closest point to the beginning of the path
distance_to_start = sqrt(sum((smoothed_path(:,closest_index) - smoothed_path(:,1)).^2));

% Calculate the distance from the closest point to the end of the path
distance_to_end = sqrt(sum((smoothed_path(:,closest_index) - smoothed_path(:,end)).^2));

% Determine the number of points to include in the instantaneous path
num_points = min(size(smoothed_path, 2), 20);

% Initialize the instantaneous_path variable using coder.nullcopy
instantaneous_path = coder.nullcopy(zeros(2, num_points));

if distance_to_start < distance_to_end
    % If the closest point is closer to the beginning of the path than the
    % end, include the points starting from the closest point towards the
    % end of the path
    start_index = closest_index;
    end_index = min(size(smoothed_path, 2), closest_index+num_points-1);
else
    % If the closest point is closer to the end of the path than the
    % beginning, include the points starting from the closest point towards
    % the beginning of the path
    start_index = max(1, closest_index-num_points+1);
    end_index = closest_index;
end

%own 
start_index = closest_index;
if start_index > 11139
    end_index = 11159;
    if start_index > 11149
        start_index = 0;
        end_index=20;
    end
else
    end_index = min(size(smoothed_path, 2), closest_index+num_points-1);
end
%own

temp_path = smoothed_path(:, start_index:end_index);
instantaneous_path(:, num_points-size(temp_path, 2)+1:num_points) = temp_path;

end

== matlab function generic_20231123_1032/CarMaker/VehicleControl/Stanley controller/MATLAB Function1 ==
  data: Pos_X input; Path_Out output; Pos_Y input; Yaw_Angle input; Path_In input
function Path_Out = Abs2RelNew(Pos_X, Pos_Y, Yaw_Angle, Path_In)
%Rotation matrix from absolute to relativ coordination system
R = [cos(Yaw_Angle) sin(Yaw_Angle); -sin(Yaw_Angle) cos(Yaw_Angle)];

Path_X=Path_In(1,:)-Pos_X;      % Shift the points in to the car position
Path_Y=Path_In(2,:)-Pos_Y;      % Shift the points in to the car position
Path=[Path_X;Path_Y];           % Car Point
Path_Out = R*Path;              % Rotate the shifted Points

== matlab function generic_20231123_1032/CarMaker/VehicleControl/Estimate object diemnsions/MATLAB Function ==
  data: range input; estimatedWidth output; azimuth input; elevation input; sensorFOV input; estimatedHeight output; sensorHeight input
function [estimatedWidth, estimatedHeight] = estimateObjectDimensions(range, azimuth, elevation, sensorFOV, sensorHeight)
    % Estimate object dimensions based on perspective projection

    % Assuming sensorFOV is in degrees
    sensorFOV_horizontal = deg2rad(sensorFOV(1));
    sensorFOV_vertical = deg2rad(sensorFOV(2));

    % Adjusted width and height based on perspective projection
    adjustedWidth =  range * tan(sensorFOV_horizontal / 2);
    adjustedHeight =   range * tan(sensorFOV_vertical / 2);

    % Adjust dimensions based on azimuth and elevation
    % For simplicity, assuming azimuth and elevation are angles in radians
    % You may need to adjust based on your sensor's coordinate system

    % Width adjustment based on azimuth
    adjustedWidth = adjustedWidth * cos(azimuth*22.5);

    % Height adjustment based on elevation
    adjustedHeight = adjustedHeight * cos(elevation*22.5);

    % Correct for perspective distortion based on sensor height
   % if sensorHeight > 0
        %perspectiveFactor = sensorHeight / range;
        %adjustedWidth = adjustedWidth * perspectiveFactor;
        %adjustedHeight = adjustedHeight * perspectiveFactor;
  %end

    estimatedWidth = adjustedWidth;
    estimatedHeight = adjustedHeight;
end

== matlab function generic_20231123_1032/CarMaker/VehicleControl/CreateBus VhclCtrl/Subsystem4/MATLAB Function6 ==
  data: path_dev input; error output; y_dev input; y_error3 input; y_error_2 input; y_error input; distance input; x_distance_obj input
function error= fcn(path_dev, y_dev, y_error3, y_error_2, y_error, distance, x_distance_obj)
if distance <15 && distance >1
    %if y_error >0 || y_error_2 >0 || y_error3 >0
    %error =-(path_dev+y_dev/2);
    %else
        error =path_dev-y_dev/2;
elseif distance <1 && distance >-4
    error =path_dev/4-y_dev/2;
elseif (distance <-5 && distance >-8) && x_distance_obj >0
    error = -path_dev/4;
elseif distance <-6 && distance >-11.5
    error = -path_dev + path_dev/1.69; % path_dev - something_ (positve->0 when the we are not near the object
else
    error = path_dev;
end
end

== matlab function generic_20231123_1032/CarMaker/VehicleControl/CreateBus VhclCtrl/Subsystem4/MATLAB Function8 ==
  data: y_added output; y_dev input; data input; distance input
function y_added= fcn( y_dev, data, distance)
if distance <12 && distance >-4
   y_added = data+y_dev;
else
    y_added = 0;
end
end

== matlab function generic_20231123_1032/CarMaker/VehicleControl/CreateBus VhclCtrl/MATLAB Function1 ==
  data: e input; steering output; Cf input; Cr input; v input
function steering = fcn(e,Cf,Cr,v)
%lf = 1.488
%lr = 1.487;
%Cf = 
%Cr =
%m =
% v = 
steering = ((lf+lr)- (lf*Cf-lr*Cr)*m*vx^2)*e...
    /(d_pre*(d_pre+2*L));

== matlab function generic_20231123_1032/CarMaker/VehicleControl/CreateBus VhclCtrl/path_planner_MATLAB/MATLAB Function1 ==
  data: u input; path_x output; path_y output; path_yaw output
function [path_x,path_y,path_yaw] = fcn(u)
path_x = u(1,:);
path_y = u(2,:);
path_yaw = u(3,:);
end

== matlab function generic_20231123_1032/CarMaker/VehicleControl/CreateBus VhclCtrl/path_planner_MATLAB/MATLAB Function ==
  data: path input; e output; yaw input; speed_act input; err_fr_axle output; cross_track_steering output; heading_err output; steering output
function [e, err_fr_axle, cross_track_steering, heading_err, steering]  = conversion(path,yaw,speed_act)
%path = [path_x;path_y];
function distance = calc_distance(pt,v1,v2)
    vect = v1 - v2;
    p_to_vect = pt - v2;
    crossVP = cross(vect,p_to_vect);
    distance = norm(crossVP) / norm(vect) * crossVP(3)/abs(crossVP(3));
end

e = zeros(1);
cross_track_steering = zeros(1);
heading_err = zeros(1);
steering=zeros(1);
err_fr_axle = zeros(1);

k_exp = 1.36;
k_def = 6;
k = k_def + abs(speed_act)^k_exp;
k_ref = 3.1;

% path_index = fix(k_path * speed_act);
% if path_index > 13
%     path_index = 13;
% end
% 
% P_prev = path(:,6 + path_index);
% P_next = path(:,7 + path_index);

fr_axle = [-1.488 0 0];
distances = sqrt((path(1,:) - 1.488).^2 + (path(2,:) - 0).^2);
% Find the index of the closest point on the path
[~,err_fr_axle_ind] = min(distances);
if err_fr_axle_ind == 1
    err_fr_axle_ind = 2;
end
err_fr_axle = calc_distance(fr_axle,[path(1,err_fr_axle_ind - 1) path(2,err_fr_axle_ind - 1) 0],[path(1,err_fr_axle_ind) path(2,err_fr_axle_ind) 0]);

B = [-1.488 + k_ref * (speed_act / 27) 0 0];
distances_err = sqrt((path(1,:) - B(1)).^2 + (path(2,:) - 0).^2);
[~,err_ind] = min(distances_err);
if err_ind < 2
    err_ind = 2;
end
error = calc_distance(B,[path(1,err_ind - 1) path(2,err_ind - 1) 0],[path(1,err_ind) path(2,err_ind) 0]);


P_prev = path(:, err_ind-1);
P_next = path(:, err_ind);

x1 = P_prev(1,1);
y1 = P_prev(2,1);
x2 = P_next(1,1);
y2 = P_next(2,1);

a = (y2 - y1)/-(x2 + x1);
b = 1;
%c = -x1 * (y2 - y1) + y1 * (x2 - x1);


if speed_act ~= 0
    %e = c+b*y1/sqrt((a^2)+(b^2));
    e = error;
    
    cross_track_steering = atan(k * e / speed_act);
    heading_err = atan(-a / b) - yaw;
    %heading_err = 1/(tan(-a/b))-yaw;
    steering = heading_err + cross_track_steering;
end
end

== matlab function generic_20231123_1032/CarMaker/VehicleControl/CreateBus VhclCtrl/path_planner_MATLAB/MATLAB Function2 ==
  data: Pos_X input; Path_Out output; Pos_Y input; Yaw_Angle input; Path_In input
function Path_Out = Abs2RelNew(Pos_X, Pos_Y, Yaw_Angle, Path_In)
%Rotation matrix from absolute to relativ coordination system
R = [cos(Yaw_Angle) sin(Yaw_Angle); -sin(Yaw_Angle) cos(Yaw_Angle)];

Path_X=Path_In(1,:)-Pos_X;      % Shift the points in to the car position
Path_Y=Path_In(2,:)-Pos_Y;      % Shift the points in to the car position
Path=[Path_X;Path_Y];           % Car Point
Path_Out = R*Path;              % Rotate the shifted Points

== matlab function generic_20231123_1032/CarMaker/VehicleControl/CreateBus VhclCtrl.Steering/MATLAB Function1 ==
  data: dev_dest input; error output; y_car input; Y_dev input
function error = fcn(dev_dest, y_car, Y_dev)
if y_car <10 && y_car>0
    error = -y_car;

else
    error =dev_dest;
end
end

== matlab function generic_20231123_1032/CarMaker/VehicleControl/CreateBus VhclCtrl/path_planner_MATLAB/Path_Calculation_V02 ==
  data: x_car input; closest_point output; y_car input; path_x input; instantaneous_path output; y_path input
function [closest_point, instantaneous_path] = calculate_path(x_car, y_car, path_x, y_path)
% x_car: x position of the car
% y_car: y position of the car
% path: [2x400] matrix representing the path
path = [path_x;y_path];
%Smoothing the Path
x = path(1,:);
y = path(2,:);
% Define the number of points you want to add for interpolation
num_extra_points = 0; % Adjust this value as per your requirements
% Compute the total number of points after interpolation
total_points = numel(x) + num_extra_points;
existing_indices = 1:numel(x);
% Create an array of indices for the interpolated points
interpolated_indices = linspace(1, numel(x), total_points);
% Perform spline interpolation on both x and y coordinates
x_interpolated = spline(existing_indices, x, interpolated_indices);
y_interpolated = spline(existing_indices, y, interpolated_indices);

smoothed_path =vertcat(x_interpolated, y_interpolated);
% smoothed_path = smoothed_path_t';


% Calculate the distance between the car and each point on the path
distances = sqrt((smoothed_path(1,:) - x_car).^2 + (smoothed_path(2,:) - y_car).^2);

% Find the index of the closest point on the path
[~, closest_index] = min(distances);

% Get the closest point on the path
closest_point = smoothed_path(:, closest_index);

% Calculate the distance from the closest point to the beginning of the path
distance_to_start = sqrt(sum((smoothed_path(:,closest_index) - smoothed_path(:,1)).^2));

% Calculate the distance from the closest point to the end of the path
distance_to_end = sqrt(sum((smoothed_path(:,closest_index) - smoothed_path(:,end)).^2));

% Determine the number of points to include in the instantaneous path
num_points = min(size(smoothed_path, 2), 20);

% Initialize the instantaneous_path variable using coder.nullcopy
instantaneous_path = coder.nullcopy(zeros(2, num_points));

if distance_to_start < distance_to_end
    % If the closest point is closer to the beginning of the path than the
    % end, include the points starting from the closest point towards the
    % end of the path
    start_index = closest_index;
    end_index = min(size(smoothed_path, 2), closest_index+num_points-1);
else
    % If the closest point is closer to the end of the path than the
    % beginning, include the points starting from the closest point towards
    % the beginning of the path
    start_index = max(1, closest_index-num_points+1);
    end_index = closest_index;
end

%own 
start_index = closest_index;
if start_index > 11139
    end_index = 11159;
    if start_index > 11149
        start_index = 0;
        end_index=20;
    end
else
    end_index = min(size(smoothed_path, 2), closest_index+num_points-1);
end
%own

temp_path = smoothed_path(:, start_index:end_index);
instantaneous_path(:, num_points-size(temp_path, 2)+1:num_points) = temp_path;

end
